simulink library "actuators_lib"  (R2016b)
settings: Solver=ode45  StartTime=0.0  StopTime=10.0  RelTol=1e-3  EnableMultiTasking=on
undefined symbols (not defined in the file or in its folder): MT_pwr, MT_valid
libraries: bus_stubs_template x2, magnetorquer_assembly_lib x1
settings Model: Creator=bbarz_000  LastModifiedBy=Taylor
settings DataIOCC: LimitDataPoints=on
settings OptimizationCC: LifeSpan=inf
settings DebuggingCC: AllowSymbolicDim=off  SFUnexpectedBacktrackingDiag=warning  SFNoUnconditionalDefaultTransitionDiag=warning  SFExecutionAtInitializationDiag=none
settings GRTTargetCC: TargetLangStandard=C89/C90 (ANSI)  GeneratePreprocessorConditionals=Disable all
settings ConfigComp: CovMetricSettings=dw  CovHtmlReporting=on  CovSaveCumulativeToWorkspaceVar=on  CovSaveSingleToWorkspaceVar=on  CovExternalEMLEnable=off

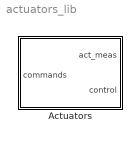
== system actuators_lib ==
  Actuators : Subsystem

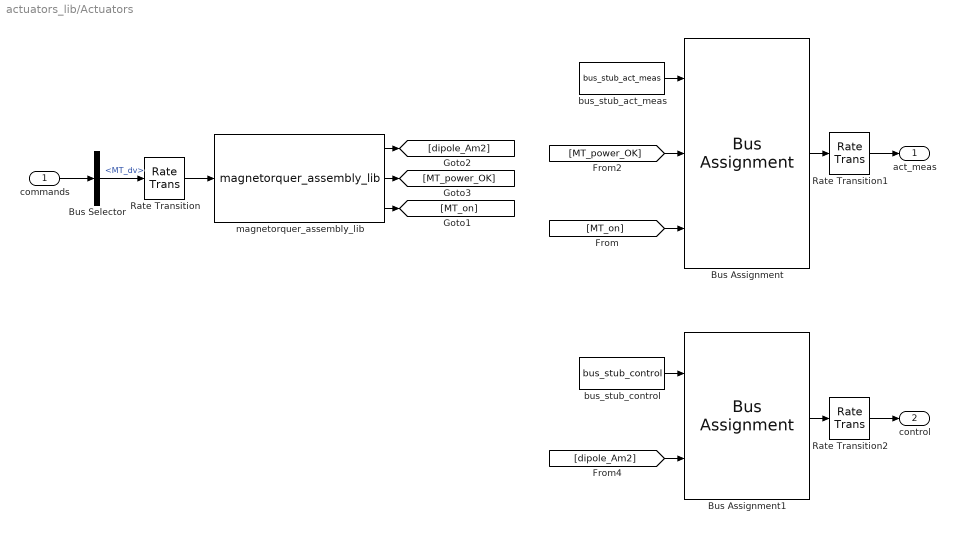
== system actuators_lib/Actuators ==
  commands : Inport  OutDataTypeStr=Bus: commands
  Bus Assignment : BusAssignment  AssignedSignals=MT_valid,MT_pwr
  Bus Assignment1 : BusAssignment  AssignedSignals=MT_dipole_Am2
  Bus Selector : BusSelector  OutputSignals=MT_dv
  Rate Transition : RateTransition  OutPortSampleTime=sim_params.sample_time_s
  Rate Transition1 : RateTransition
  Rate Transition2 : RateTransition
  bus_stub_act_meas : bus_stubs_template/bus_stub_act_meas
  bus_stub_control : bus_stubs_template/bus_stub_control
  magnetorquer_assembly_lib : magnetorquer_assembly_lib/magnetorquer_assembly_lib
  act_meas : Outport
  control : Outport  Port=2
  wires:
  commands/1 -> Bus Selector/1
  Bus Assignment/1 -> Rate Transition1/1
  bus_stub_act_meas/1 -> Bus Assignment/1
  bus_stub_control/1 -> Bus Assignment1/1
  Bus Assignment1/1 -> Rate Transition2/1
  Bus Selector/1 -> Rate Transition/1  "<MT_dv>"
  magnetorquer_assembly_lib/1 -> [dipole_Am2]
  magnetorquer_assembly_lib/2 -> [MT_power_OK]
  magnetorquer_assembly_lib/3 -> [MT_on]
  [MT_power_OK] -> Bus Assignment/2
  [dipole_Am2] -> Bus Assignment1/2
  [MT_on] -> Bus Assignment/3
  Rate Transition/1 -> magnetorquer_assembly_lib/1
  Rate Transition1/1 -> act_meas/1
  Rate Transition2/1 -> control/1
